simulink model "mobile3"  (R2022b)
settings: Solver=VariableStepAuto  StartTime=0.0  StopTime=10.0  RelTol=1e-3
settings Model: Creator=Administrator  LastModifiedBy=Administrator
settings SolverCC: AlgebraicLoopSolver=TrustRegion
settings DataIOCC: ReturnWorkspaceOutputs=off
settings DebuggingCC: UnconnectedInputMsg=warning  UnconnectedOutputMsg=warning  UnconnectedLineMsg=warning  SFMachineParentedDataDiag=warning  ArithmeticOperatorsInVariantConditions=warning
settings ModelReferenceCC: EnableRefExpFcnMdlSchedulingChecks=on
settings SFSimCC: SimUseLocalCustomCode=off  CustomCodeUndefinedFunction=UseInterfaceOnly
settings RTWCC: RTWUseLocalCustomCode=off

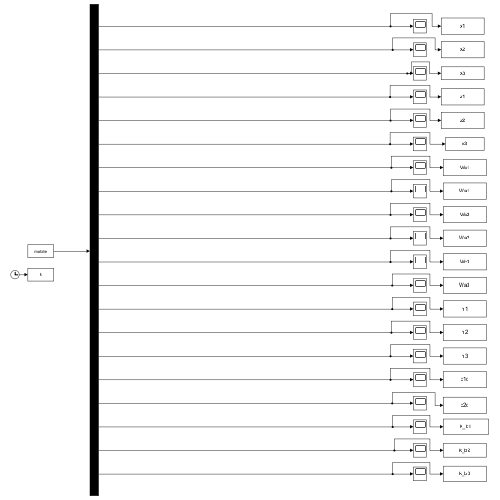
[thumbnail: Simulink's stored preview of the top-level diagram]
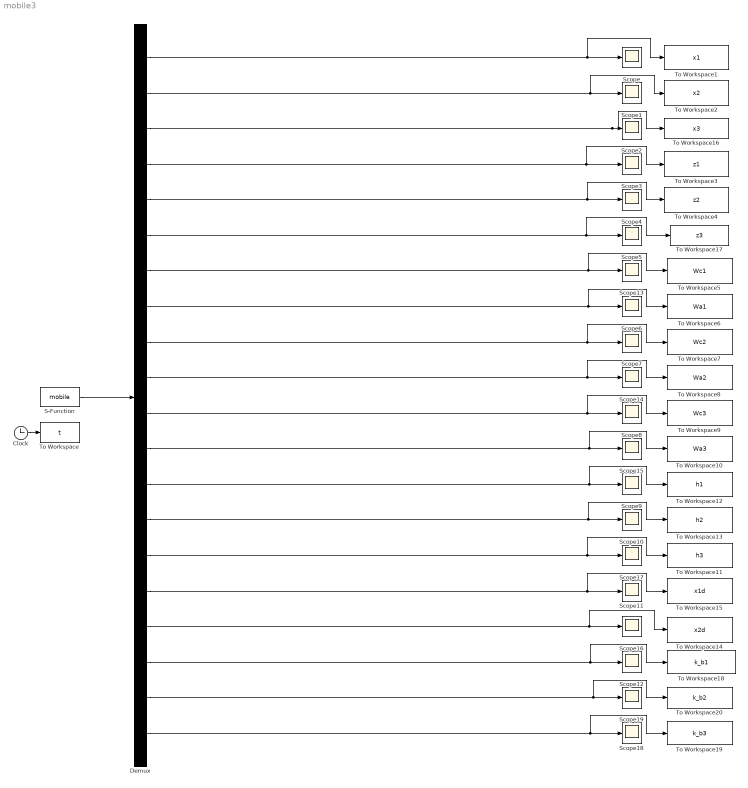
== system mobile3 ==
  Clock : Clock
  Demux : Demux  Outputs=20
  S-Function : S-Function  FunctionName=mobile  SFunctionDeploymentMode=off  EnableBusSupport=off
  Scope{,1..19} (20 alike) : Scope
  To Workspace : ToWorkspace  VariableName=t  SaveFormat=Timeseries  SampleTime=-1
  To Workspace1 : ToWorkspace  VariableName=x1  SaveFormat=Timeseries  SampleTime=-1
  To Workspace10 : ToWorkspace  VariableName=Wa3  SaveFormat=Timeseries  SampleTime=-1
  To Workspace11 : ToWorkspace  VariableName=h3  SaveFormat=Timeseries  SampleTime=-1
  To Workspace12 : ToWorkspace  VariableName=h1  SaveFormat=Timeseries  SampleTime=-1
  To Workspace13 : ToWorkspace  VariableName=h2  SaveFormat=Timeseries  SampleTime=-1
  To Workspace14 : ToWorkspace  VariableName=x2d  SaveFormat=Timeseries  SampleTime=-1
  To Workspace15 : ToWorkspace  VariableName=x1d  SaveFormat=Timeseries  SampleTime=-1
  To Workspace16 : ToWorkspace  VariableName=x3  SaveFormat=Timeseries  SampleTime=-1
  To Workspace17 : ToWorkspace  VariableName=z3  SaveFormat=Timeseries  SampleTime=-1
  To Workspace18 : ToWorkspace  VariableName=k_b1  SaveFormat=Timeseries  SampleTime=-1
  To Workspace19 : ToWorkspace  VariableName=k_b3  SaveFormat=Timeseries  SampleTime=-1
  To Workspace2 : ToWorkspace  VariableName=x2  SaveFormat=Timeseries  SampleTime=-1
  To Workspace20 : ToWorkspace  VariableName=k_b2  SaveFormat=Timeseries  SampleTime=-1
  To Workspace3 : ToWorkspace  VariableName=z1  SaveFormat=Timeseries  SampleTime=-1
  To Workspace4 : ToWorkspace  VariableName=z2  SaveFormat=Timeseries  SampleTime=-1
  To Workspace5 : ToWorkspace  VariableName=Wc1  SaveFormat=Timeseries  SampleTime=-1
  To Workspace6 : ToWorkspace  VariableName=Wa1  SaveFormat=Timeseries  SampleTime=-1
  To Workspace7 : ToWorkspace  VariableName=Wc2  SaveFormat=Timeseries  SampleTime=-1
  To Workspace8 : ToWorkspace  VariableName=Wa2  SaveFormat=Timeseries  SampleTime=-1
  To Workspace9 : ToWorkspace  VariableName=Wc3  SaveFormat=Timeseries  SampleTime=-1
  wires:
  Clock/1 -> To Workspace/1
  S-Function/1 -> Demux/1
  Demux/2 -> To Workspace2/1, Scope1/1
  Demux/3 -> To Workspace16/1, Scope2/1
  Demux/4 -> To Workspace3/1, Scope3/1
  Demux/5 -> To Workspace4/1, Scope4/1
  Demux/6 -> To Workspace17/1, Scope5/1
  Demux/7 -> To Workspace5/1, Scope13/1
  Demux/8 -> To Workspace6/1, Scope6/1
  Demux/9 -> To Workspace7/1, Scope7/1
  Demux/10 -> To Workspace8/1, Scope14/1
  Demux/11 -> To Workspace9/1, Scope8/1
  Demux/12 -> To Workspace10/1, Scope15/1
  Demux/13 -> To Workspace12/1, Scope9/1
  Demux/14 -> To Workspace13/1, Scope10/1
  Demux/15 -> To Workspace11/1, Scope17/1
  Demux/16 -> To Workspace15/1, Scope11/1
  Demux/17 -> To Workspace14/1, Scope16/1
  Demux/18 -> To Workspace18/1, Scope12/1
  Demux/19 -> To Workspace20/1, Scope19/1
  Demux/20 -> To Workspace19/1, Scope18/1
  Demux/1 -> To Workspace1/1, Scope/1
